simulink model "wrench_maats_simulator_v3"  (R2025b)
settings: Solver=ode15s  StartTime=0.0  StopTime=100  FixedStep=1e-4  RelTol=1e-3
values from neighbouring files (symbols this model uses):
  Kd1 = 2    [parametrosCarga4x.m]
  x1_0 = xL0+q1_rot*[0;0;L1]    [parametrosCarga4x.m]
  x2_0 = xL0+q2_rot*[0;0;L2]    [parametrosCarga4x.m]
  x3_0 = xL0+q3_rot*[0;0;L3]    [parametrosCarga4x.m]
  x4_0 = xL0+q4_rot*[0;0;L4]    [parametrosCarga4x.m]
settings Model: Creator=ateveraz  LastModifiedBy=ateveraz

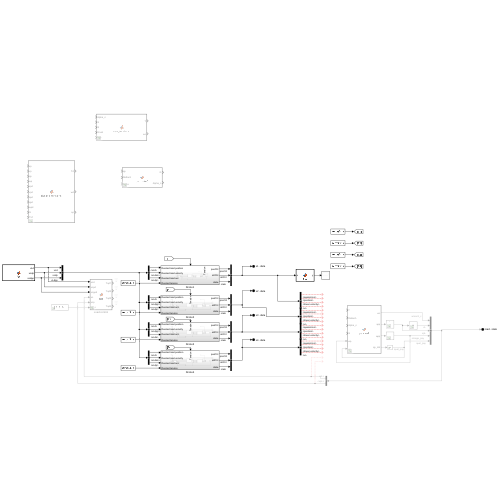
[thumbnail: Simulink's stored preview of the top-level diagram]
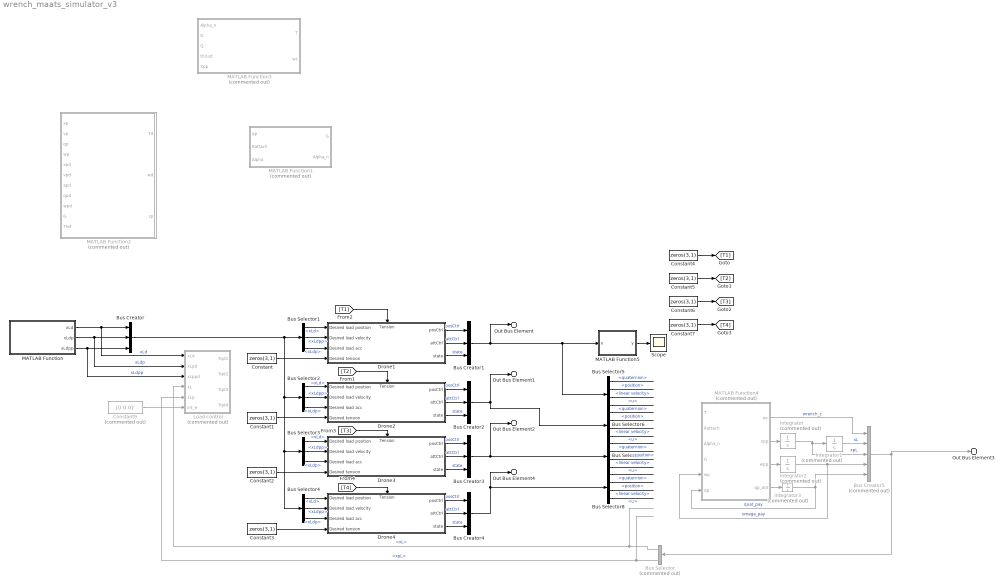
== system wrench_maats_simulator_v3 ==
  Bus Creator{,2..4} (4 alike) : BusCreator  Inputs=3
  Bus Creator1 : BusCreator  Inputs=3  OutDataTypeStr=Bus: busx1
  Bus Creator5 : BusCreator  Commented=on  Inputs=5
  Bus Selector : BusSelector  Commented=on  OutputSignals=xL,xpL
  Bus Selector{1..4} (4 alike) : BusSelector  OutputSignals=xLd,xLdpp,xLdp
  Bus Selector{5..8} (4 alike) : BusSelector  OutputSignals=state.quaternion,state.position,state.linear velocity,posCtrl.u
  Constant{,1..7} (8 alike) : Constant  Value=zeros(3,1)
  Constant9 : Constant  Commented=on  Value=[0 0 0]'
  Drone1 : Subsystem
      settings: PortSchema="{\"entries\":[{\"content\":{\"sides\":[{\"content\":{\"connectorIds\":[\"In1\",\"In2\",\"In3\",\"In4\"]},\"type\":\"ConnectorPlacement.EquallySpacedRectSide\",\"uuid\":\"21103dfc-7bbe-40e0-9fc6-037905f1ea97\"},{\"content\":{\"connectorIds\":[\"Out1\",\"Out2\",\"Out3\"],\"side\":\"RIGHT\"},\"type\":\"ConnectorPlacement.EquallySpacedRectSide\",\"uuid\":\"5db0cf3b-93f2-491f-9cf6-07daf4674486\"},{\"content\":{\"connectorIds\":[\"In5\"],\"side\":\"TOP\"},\"type\":\"ConnectorPlacement.EquallySpacedRectSide\",\"uuid\":\"a4b55797-f354-4dcd-9bd0-022aba8efa3f\"}]},\"type\":\"ConnectorPlacement.EquallySpacedConnector\",\"uuid\":\"4e7ed67a-de76-4120-bfce-551a78690751\"}],\"packageUris\":[\"http://schema.mathworks.com/mf0/Connector/R2020b\"],\"version\":\"1.0\"}"
  Drone2 : Subsystem
      settings: PortSchema="{\"entries\":[{\"content\":{\"sides\":[{\"content\":{\"connectorIds\":[\"In1\",\"In2\",\"In3\",\"In4\"]},\"type\":\"ConnectorPlacement.EquallySpacedRectSide\",\"uuid\":\"21103dfc-7bbe-40e0-9fc6-037905f1ea97\"},{\"content\":{\"connectorIds\":[\"Out1\",\"Out2\",\"Out3\"],\"side\":\"RIGHT\"},\"type\":\"ConnectorPlacement.EquallySpacedRectSide\",\"uuid\":\"5db0cf3b-93f2-491f-9cf6-07daf4674486\"},{\"content\":{\"connectorIds\":[\"In5\"],\"side\":\"TOP\"},\"type\":\"ConnectorPlacement.EquallySpacedRectSide\",\"uuid\":\"a4b55797-f354-4dcd-9bd0-022aba8efa3f\"}]},\"type\":\"ConnectorPlacement.EquallySpacedConnector\",\"uuid\":\"4e7ed67a-de76-4120-bfce-551a78690751\"}],\"packageUris\":[\"http://schema.mathworks.com/mf0/Connector/R2020b\"],\"version\":\"1.0\"}"
  Drone3 : Subsystem
      settings: PortSchema="{\"entries\":[{\"content\":{\"sides\":[{\"content\":{\"connectorIds\":[\"In1\",\"In2\",\"In3\",\"In4\"]},\"type\":\"ConnectorPlacement.EquallySpacedRectSide\",\"uuid\":\"21103dfc-7bbe-40e0-9fc6-037905f1ea97\"},{\"content\":{\"connectorIds\":[\"Out1\",\"Out2\",\"Out3\"],\"side\":\"RIGHT\"},\"type\":\"ConnectorPlacement.EquallySpacedRectSide\",\"uuid\":\"5db0cf3b-93f2-491f-9cf6-07daf4674486\"},{\"content\":{\"connectorIds\":[\"In5\"],\"side\":\"TOP\"},\"type\":\"ConnectorPlacement.EquallySpacedRectSide\",\"uuid\":\"a4b55797-f354-4dcd-9bd0-022aba8efa3f\"}]},\"type\":\"ConnectorPlacement.EquallySpacedConnector\",\"uuid\":\"4e7ed67a-de76-4120-bfce-551a78690751\"}],\"packageUris\":[\"http://schema.mathworks.com/mf0/Connector/R2020b\"],\"version\":\"1.0\"}"
  Drone4 : Subsystem
      settings: PortSchema="{\"entries\":[{\"content\":{\"sides\":[{\"content\":{\"connectorIds\":[\"In1\",\"In2\",\"In3\",\"In4\"]},\"type\":\"ConnectorPlacement.EquallySpacedRectSide\",\"uuid\":\"21103dfc-7bbe-40e0-9fc6-037905f1ea97\"},{\"content\":{\"connectorIds\":[\"Out1\",\"Out2\",\"Out3\"],\"side\":\"RIGHT\"},\"type\":\"ConnectorPlacement.EquallySpacedRectSide\",\"uuid\":\"5db0cf3b-93f2-491f-9cf6-07daf4674486\"},{\"content\":{\"connectorIds\":[\"In5\"],\"side\":\"TOP\"},\"type\":\"ConnectorPlacement.EquallySpacedRectSide\",\"uuid\":\"a4b55797-f354-4dcd-9bd0-022aba8efa3f\"}]},\"type\":\"ConnectorPlacement.EquallySpacedConnector\",\"uuid\":\"4e7ed67a-de76-4120-bfce-551a78690751\"}],\"packageUris\":[\"http://schema.mathworks.com/mf0/Connector/R2020b\"],\"version\":\"1.0\"}"
  Integrator{,1..3} (4 alike) : Integrator  Commented=on
  Load control : MATLAB Function  Commented=on  TreatAsAtomicUnit=on
  MATLAB Function : MATLAB Function  TreatAsAtomicUnit=on
  MATLAB Function1 : MATLAB Function  Commented=on  TreatAsAtomicUnit=on
  MATLAB Function2 : MATLAB Function  Commented=on  TreatAsAtomicUnit=on
  MATLAB Function3 : MATLAB Function  Commented=on  TreatAsAtomicUnit=on
  MATLAB Function4 : MATLAB Function  Commented=on  TreatAsAtomicUnit=on
  MATLAB Function5 : MATLAB Function  TreatAsAtomicUnit=on
  Scope : Scope
  Out Bus Element3 : Outport  PortName=load  Element=state
  Out Bus Element : Outport  Port=2  PortName=x1  Element=data
  Out Bus Element1 : Outport  Port=3  PortName=x2  Element=data
  Out Bus Element2 : Outport  Port=4  PortName=x3  Element=data
  Out Bus Element4 : Outport  Port=5  PortName=x4  Element=data
  wires:
  Drone1/1(posCtrl) -> Bus Creator1/1  "posCtrl"
  Drone1/2(attCtrl) -> Bus Creator1/2  "attCtrl"
  Drone1/3(state) -> Bus Creator1/3  "state"
  MATLAB Function/1(xLd) -> Load control/1(xLd), Bus Creator/1  "xLd"
  MATLAB Function/2(xLdp) -> Load control/2(xLpd), Bus Creator/2  "xLdp"
  MATLAB Function/3(xLdpp) -> Load control/3(xLppd), Bus Creator/3  "xLdpp"
  Constant9/1 -> Load control/6(int_e)
  Bus Creator5/1 -> Out Bus Element3/1, Bus Selector/1
  Bus Selector/2 -> Load control/5(xLp)  "<xpL>"
  Bus Selector/1 -> Load control/4(xL)  "<xL>"
  Bus Selector1/1 -> Drone1/1(Desired load position)  "<xLd>"
  Bus Selector1/2 -> Drone1/2(Desired load velocity)  "<xLdpp>"
  Bus Selector1/3 -> Drone1/3(Desired load acc)  "<xLdp>"
  Bus Selector2/3 -> Drone2/3(Desired load acc)  "<xLdp>"
  Bus Selector2/2 -> Drone2/2(Desired load velocity)  "<xLdpp>"
  Bus Selector2/1 -> Drone2/1(Desired load position)  "<xLd>"
  Bus Creator/1 -> Bus Selector4/1, Bus Selector3/1, Bus Selector2/1, Bus Selector1/1
  Bus Selector3/2 -> Drone3/2(Desired load velocity)  "<xLdpp>"
  Bus Selector3/3 -> Drone3/3(Desired load acc)  "<xLdp>"
  Bus Selector3/1 -> Drone3/1(Desired load position)  "<xLd>"
  Bus Selector4/1 -> Drone4/1(Desired load position)  "<xLd>"
  Bus Selector4/3 -> Drone4/3(Desired load acc)  "<xLdp>"
  Bus Selector4/2 -> Drone4/2(Desired load velocity)  "<xLdpp>"
  Bus Creator1/1 -> MATLAB Function5/1(u), Bus Selector5/1, Out Bus Element/1
  Bus Creator2/1 -> Out Bus Element1/1, Bus Selector6/1
  Drone2/3(state) -> Bus Creator2/3  "state"
  Drone2/2(attCtrl) -> Bus Creator2/2  "attCtrl"
  Drone2/1(posCtrl) -> Bus Creator2/1  "posCtrl"
  Drone3/1(posCtrl) -> Bus Creator3/1  "posCtrl"
  Drone3/2(attCtrl) -> Bus Creator3/2  "attCtrl"
  Drone3/3(state) -> Bus Creator3/3  "state"
  Bus Creator3/1 -> Out Bus Element2/1, Bus Selector7/1
  Bus Creator4/1 -> Bus Selector8/1, Out Bus Element4/1
  Drone4/3(state) -> Bus Creator4/3  "state"
  Drone4/2(attCtrl) -> Bus Creator4/2  "attCtrl"
  Drone4/1(posCtrl) -> Bus Creator4/1  "posCtrl"
  Bus Selector5/1 -> ?  "<quaternion>"
  Bus Selector5/2 -> ?  "<position>"
  Bus Selector5/3 -> ?  "<linear velocity>"
  Bus Selector5/4 -> ?  "<u>"
  Bus Selector6/1 -> ?  "<quaternion>"
  Bus Selector6/2 -> ?  "<position>"
  Bus Selector6/3 -> ?  "<linear velocity>"
  Bus Selector6/4 -> ?  "<u>"
  Bus Selector7/1 -> ?  "<quaternion>"
  Bus Selector7/2 -> ?  "<position>"
  Bus Selector7/3 -> ?  "<linear velocity>"
  Bus Selector7/4 -> ?  "<u>"
  Bus Selector8/1 -> ?  "<quaternion>"
  Bus Selector8/2 -> ?  "<position>"
  Bus Selector8/3 -> ?  "<linear velocity>"
  Bus Selector8/4 -> ?  "<u>"
  [T2] -> Drone2/5(Tension)
  [T3] -> Drone3/5(Tension)
  [T4] -> Drone4/5(Tension)
  [T1] -> Drone1/5(Tension)
  Integrator/1 -> Bus Creator5/3, Integrator1/1  "xpL"
  MATLAB Function4/3(wpp) -> Integrator2/1
  Integrator2/1 -> Bus Creator5/4, MATLAB Function4/5(wp)  "omega_pay"
  MATLAB Function4/4(qp_dot) -> Integrator3/1
  Integrator3/1 -> MATLAB Function4/6(qp), Bus Creator5/5  "quat_pay"
  MATLAB Function4/2(xpp) -> Integrator/1
  Integrator1/1 -> Bus Creator5/2  "xL"
  MATLAB Function4/1(wc) -> Bus Creator5/1  "wrench_c"
  Constant/1 -> Drone1/4(Desired tension)
  Constant1/1 -> Drone2/4(Desired tension)
  Constant2/1 -> Drone3/4(Desired tension)
  Constant3/1 -> Drone4/4(Desired tension)
  Constant4/1 -> [T1]
  Constant5/1 -> [T2]
  Constant6/1 -> [T3]
  Constant7/1 -> [T4]
  MATLAB Function5/1(y) -> Scope/1

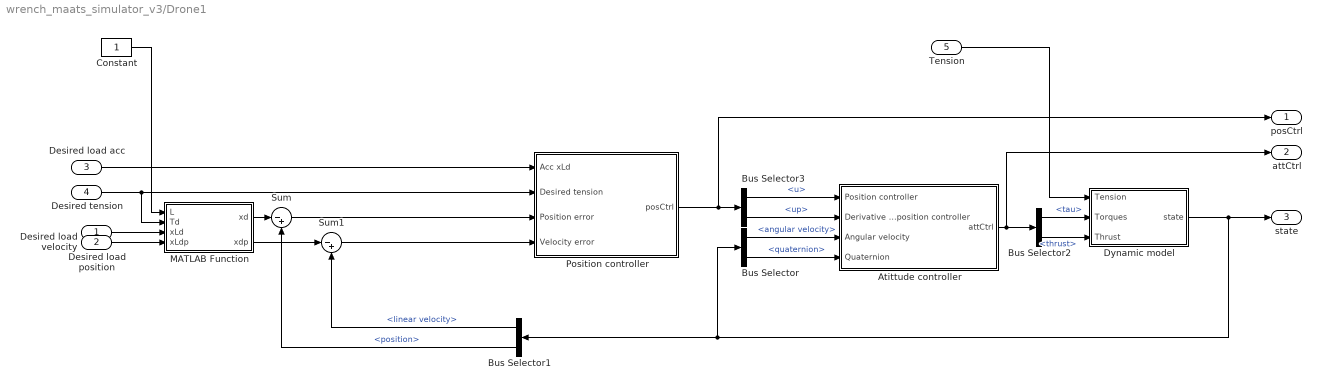
== system wrench_maats_simulator_v3/Drone1 ==
  Desired load position : Inport
  Desired load velocity : Inport  Port=2
  Desired load acc : Inport  Port=3
  Desired tension : Inport  Port=4
  Tension : Inport  Port=5
  Atittude controller : Subsystem
  Bus Selector : BusSelector  OutputSignals=angular velocity,quaternion
  Bus Selector1 : BusSelector  OutputSignals=linear velocity,position
  Bus Selector2 : BusSelector  OutputSignals=tau,thrust
  Bus Selector3 : BusSelector  OutputSignals=u,up
  Constant : Constant
  Dynamic model : Subsystem
  MATLAB Function : MATLAB Function  TreatAsAtomicUnit=on
  Position controller : Subsystem
  Sum : Sum  Inputs=|-+
  Sum1 : Sum  Inputs=|-+
  posCtrl : Outport
  attCtrl : Outport  Port=2
  state : Outport  Port=3
  wires:
  Sum1/1 -> Position controller/4(Velocity error)
  Desired load velocity/1 -> MATLAB Function/4(xLdp)
  Bus Selector3/1 -> Atittude controller/1(Position controller)  "<u>"
  Bus Selector2/1 -> Dynamic model/2(Torques)  "<tau>"
  Atittude controller/1(attCtrl) -> attCtrl/1, Bus Selector2/1
  Desired tension/1 -> MATLAB Function/2(Td), Position controller/2(Desired tension)
  Desired load acc/1 -> Position controller/1(Acc xLd)
  Sum/1 -> Position controller/3(Position error)
  Bus Selector1/2 -> Sum/2  "<position>"
  Position controller/1(posCtrl) -> posCtrl/1, Bus Selector3/1
  Bus Selector2/2 -> Dynamic model/3(Thrust)  "<thrust>"
  Desired load position/1 -> MATLAB Function/3(xLd)
  Bus Selector1/1 -> Sum1/2  "<linear velocity>"
  Dynamic model/1(state) -> Bus Selector/1, Bus Selector1/1, state/1
  Bus Selector3/2 -> Atittude controller/2(Derivative position controller)  "<up>"
  MATLAB Function/1(xd) -> Sum/1
  MATLAB Function/2(xdp) -> Sum1/1
  Constant/1 -> MATLAB Function/1(L)
  Tension/1 -> Dynamic model/1(Tension)
  Bus Selector/1 -> Atittude controller/3(Angular velocity)  "<angular velocity>"
  Bus Selector/2 -> Atittude controller/4(Quaternion)  "<quaternion>"

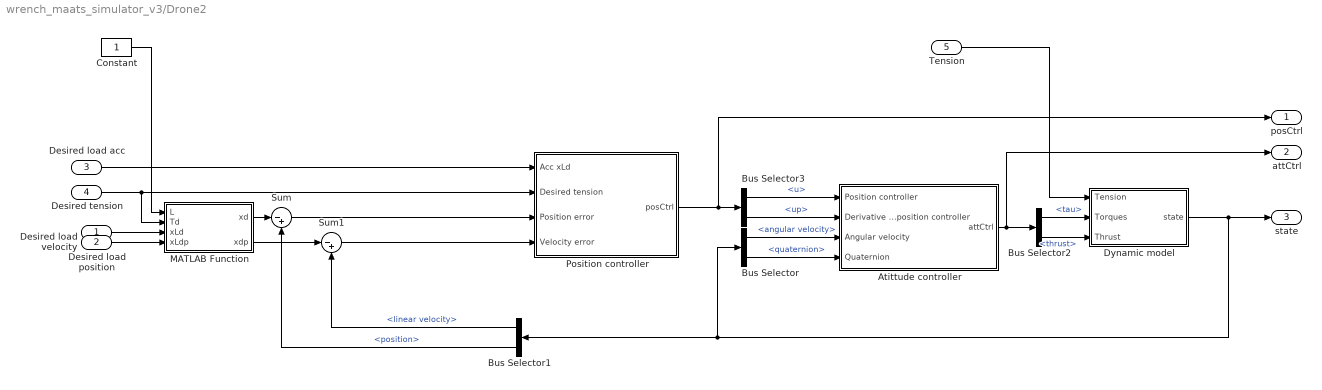
== system wrench_maats_simulator_v3/Drone2 ==
  Desired load position : Inport
  Desired load velocity : Inport  Port=2
  Desired load acc : Inport  Port=3
  Desired tension : Inport  Port=4
  Tension : Inport  Port=5
  Atittude controller : Subsystem
  Bus Selector : BusSelector  OutputSignals=angular velocity,quaternion
  Bus Selector1 : BusSelector  OutputSignals=linear velocity,position
  Bus Selector2 : BusSelector  OutputSignals=tau,thrust
  Bus Selector3 : BusSelector  OutputSignals=u,up
  Constant : Constant
  Dynamic model : Subsystem
  MATLAB Function : MATLAB Function  TreatAsAtomicUnit=on
  Position controller : Subsystem
  Sum : Sum  Inputs=|-+
  Sum1 : Sum  Inputs=|-+
  posCtrl : Outport
  attCtrl : Outport  Port=2
  state : Outport  Port=3
  wires:
  Bus Selector/2 -> Atittude controller/4(Quaternion)  "<quaternion>"
  Bus Selector/1 -> Atittude controller/3(Angular velocity)  "<angular velocity>"
  Tension/1 -> Dynamic model/1(Tension)
  Constant/1 -> MATLAB Function/1(L)
  MATLAB Function/2(xdp) -> Sum1/1
  MATLAB Function/1(xd) -> Sum/1
  Bus Selector3/2 -> Atittude controller/2(Derivative position controller)  "<up>"
  Dynamic model/1(state) -> state/1, Bus Selector1/1, Bus Selector/1
  Bus Selector1/1 -> Sum1/2  "<linear velocity>"
  Desired load position/1 -> MATLAB Function/3(xLd)
  Bus Selector2/2 -> Dynamic model/3(Thrust)  "<thrust>"
  Position controller/1(posCtrl) -> Bus Selector3/1, posCtrl/1
  Bus Selector1/2 -> Sum/2  "<position>"
  Sum/1 -> Position controller/3(Position error)
  Desired load acc/1 -> Position controller/1(Acc xLd)
  Desired tension/1 -> Position controller/2(Desired tension), MATLAB Function/2(Td)
  Atittude controller/1(attCtrl) -> Bus Selector2/1, attCtrl/1
  Bus Selector2/1 -> Dynamic model/2(Torques)  "<tau>"
  Bus Selector3/1 -> Atittude controller/1(Position controller)  "<u>"
  Desired load velocity/1 -> MATLAB Function/4(xLdp)
  Sum1/1 -> Position controller/4(Velocity error)

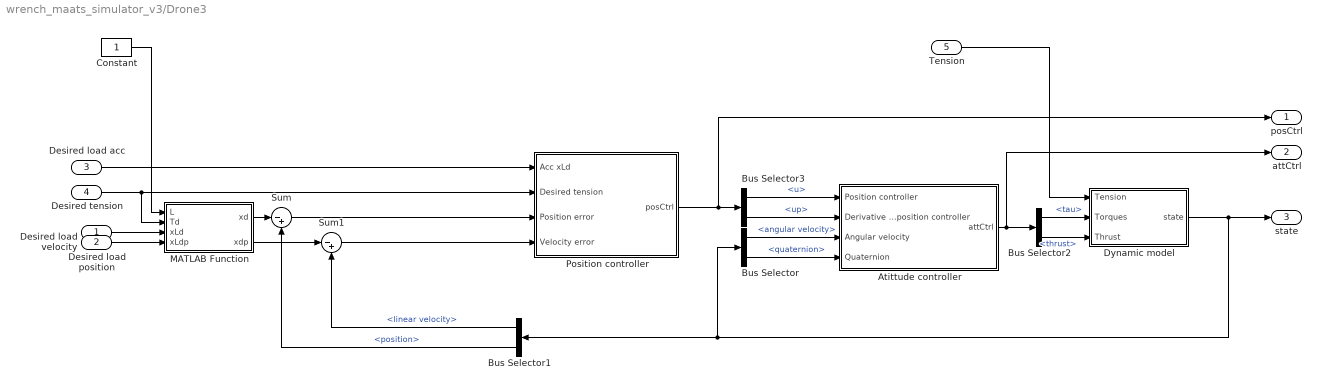
== system wrench_maats_simulator_v3/Drone3 ==
  Desired load position : Inport
  Desired load velocity : Inport  Port=2
  Desired load acc : Inport  Port=3
  Desired tension : Inport  Port=4
  Tension : Inport  Port=5
  Atittude controller : Subsystem
  Bus Selector : BusSelector  OutputSignals=angular velocity,quaternion
  Bus Selector1 : BusSelector  OutputSignals=linear velocity,position
  Bus Selector2 : BusSelector  OutputSignals=tau,thrust
  Bus Selector3 : BusSelector  OutputSignals=u,up
  Constant : Constant
  Dynamic model : Subsystem
  MATLAB Function : MATLAB Function  TreatAsAtomicUnit=on
  Position controller : Subsystem
  Sum : Sum  Inputs=|-+
  Sum1 : Sum  Inputs=|-+
  posCtrl : Outport
  attCtrl : Outport  Port=2
  state : Outport  Port=3
  wires:
  Sum1/1 -> Position controller/4(Velocity error)
  Desired load velocity/1 -> MATLAB Function/4(xLdp)
  Bus Selector3/1 -> Atittude controller/1(Position controller)  "<u>"
  Bus Selector2/1 -> Dynamic model/2(Torques)  "<tau>"
  Atittude controller/1(attCtrl) -> attCtrl/1, Bus Selector2/1
  Desired tension/1 -> MATLAB Function/2(Td), Position controller/2(Desired tension)
  Desired load acc/1 -> Position controller/1(Acc xLd)
  Sum/1 -> Position controller/3(Position error)
  Bus Selector1/2 -> Sum/2  "<position>"
  Position controller/1(posCtrl) -> posCtrl/1, Bus Selector3/1
  Bus Selector2/2 -> Dynamic model/3(Thrust)  "<thrust>"
  Desired load position/1 -> MATLAB Function/3(xLd)
  Bus Selector1/1 -> Sum1/2  "<linear velocity>"
  Dynamic model/1(state) -> Bus Selector/1, Bus Selector1/1, state/1
  Bus Selector3/2 -> Atittude controller/2(Derivative position controller)  "<up>"
  MATLAB Function/1(xd) -> Sum/1
  MATLAB Function/2(xdp) -> Sum1/1
  Constant/1 -> MATLAB Function/1(L)
  Tension/1 -> Dynamic model/1(Tension)
  Bus Selector/1 -> Atittude controller/3(Angular velocity)  "<angular velocity>"
  Bus Selector/2 -> Atittude controller/4(Quaternion)  "<quaternion>"

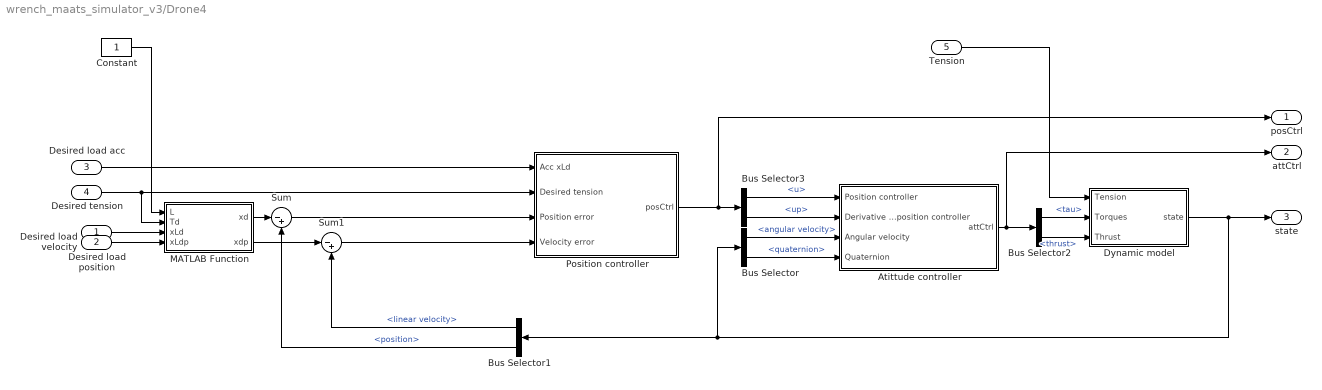
== system wrench_maats_simulator_v3/Drone4 ==
  Desired load position : Inport
  Desired load velocity : Inport  Port=2
  Desired load acc : Inport  Port=3
  Desired tension : Inport  Port=4
  Tension : Inport  Port=5
  Atittude controller : Subsystem
  Bus Selector : BusSelector  OutputSignals=angular velocity,quaternion
  Bus Selector1 : BusSelector  OutputSignals=linear velocity,position
  Bus Selector2 : BusSelector  OutputSignals=tau,thrust
  Bus Selector3 : BusSelector  OutputSignals=u,up
  Constant : Constant
  Dynamic model : Subsystem
  MATLAB Function : MATLAB Function  TreatAsAtomicUnit=on
  Position controller : Subsystem
  Sum : Sum  Inputs=|-+
  Sum1 : Sum  Inputs=|-+
  posCtrl : Outport
  attCtrl : Outport  Port=2
  state : Outport  Port=3
  wires:
  Bus Selector/2 -> Atittude controller/4(Quaternion)  "<quaternion>"
  Bus Selector/1 -> Atittude controller/3(Angular velocity)  "<angular velocity>"
  Tension/1 -> Dynamic model/1(Tension)
  Constant/1 -> MATLAB Function/1(L)
  MATLAB Function/2(xdp) -> Sum1/1
  MATLAB Function/1(xd) -> Sum/1
  Bus Selector3/2 -> Atittude controller/2(Derivative position controller)  "<up>"
  Dynamic model/1(state) -> state/1, Bus Selector1/1, Bus Selector/1
  Bus Selector1/1 -> Sum1/2  "<linear velocity>"
  Desired load position/1 -> MATLAB Function/3(xLd)
  Bus Selector2/2 -> Dynamic model/3(Thrust)  "<thrust>"
  Position controller/1(posCtrl) -> Bus Selector3/1, posCtrl/1
  Bus Selector1/2 -> Sum/2  "<position>"
  Sum/1 -> Position controller/3(Position error)
  Desired load acc/1 -> Position controller/1(Acc xLd)
  Desired tension/1 -> Position controller/2(Desired tension), MATLAB Function/2(Td)
  Atittude controller/1(attCtrl) -> Bus Selector2/1, attCtrl/1
  Bus Selector2/1 -> Dynamic model/2(Torques)  "<tau>"
  Bus Selector3/1 -> Atittude controller/1(Position controller)  "<u>"
  Desired load velocity/1 -> MATLAB Function/4(xLdp)
  Sum1/1 -> Position controller/4(Velocity error)

== system wrench_maats_simulator_v3/Drone1/Atittude controller ==
  Position controller : Inport
  Derivative position controller : Inport  Port=2
  Angular velocity : Inport  Port=3
  Quaternion : Inport  Port=4
  Bus Creator : BusCreator  Inputs=3
  MATLAB System1 : MATLABSystem  System=AttitudeController  Kd=1  beta=0.3  gamma=10  rho=18  SimulateUsing=Code generation
      mask Type: AttitudeController
  MATLAB System2 : MATLABSystem  System=DesiredAttitude  SimulateUsing=Code generation
      mask Type: DesiredAttitude
  attCtrl : Outport
  wires:
  Angular velocity/1 -> MATLAB System2/3
  MATLAB System2/2 -> MATLAB System1/3
  Position controller/1 -> MATLAB System1/1, MATLAB System2/1
  Quaternion/1 -> MATLAB System2/4
  MATLAB System2/1 -> Bus Creator/3, MATLAB System1/2  "error quaternion"
  Derivative position controller/1 -> MATLAB System2/2
  MATLAB System1/2 -> Bus Creator/2  "thrust"
  Bus Creator/1 -> attCtrl/1
  MATLAB System1/1 -> Bus Creator/1  "tau"

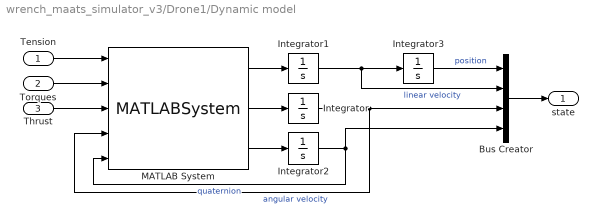
== system wrench_maats_simulator_v3/Drone1/Dynamic model ==
  Tension : Inport
  Torques : Inport  Port=2
  Thrust : Inport  Port=3
  Bus Creator : BusCreator  Inputs=4
  Integrator : Integrator  InitialCondition=[0 0 0]'
  Integrator1 : Integrator  InitialCondition=[0 0 0]'
  Integrator2 : Integrator  InitialCondition=[1 0 0 0]'
  Integrator3 : Integrator  InitialCondition=x1_0
  MATLAB System : MATLABSystem  System=Modelx4  mass=mi  inertia_matrix=J  SimulateUsing=Code generation
      mask Type: Modelx4
  state : Outport
  wires:
  MATLAB System/1 -> Integrator1/1
  Integrator3/1 -> Bus Creator/1  "position"
  MATLAB System/3 -> Integrator2/1
  MATLAB System/2 -> Integrator/1
  Integrator2/1 -> MATLAB System/5, Bus Creator/4  "quaternion"
  Torques/1 -> MATLAB System/2
  Integrator1/1 -> Bus Creator/2, Integrator3/1  "linear velocity"
  Thrust/1 -> MATLAB System/3
  Integrator/1 -> MATLAB System/4, Bus Creator/3  "angular velocity"
  Bus Creator/1 -> state/1
  Tension/1 -> MATLAB System/1

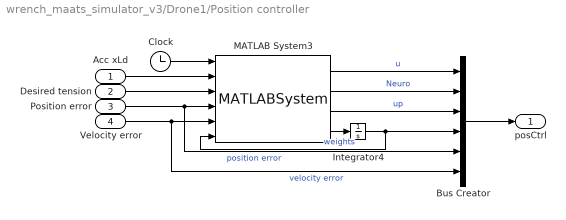
== system wrench_maats_simulator_v3/Drone1/Position controller ==
  Acc xLd : Inport
  Desired tension : Inport  Port=2
  Position error : Inport  Port=3
  Velocity error : Inport  Port=4
  Bus Creator : BusCreator  Inputs=6
  Clock : Clock
  Integrator4 : Integrator  InitialCondition=zeros(3,15)
  MATLAB System3 : MATLABSystem  System=PositionController  Kd=Kd1  alpha=Alpha1  mass=mi  Gamma=Gamma1  kappa=2  k=10  N_neurons=15  center_range=1  eta_width=linspace(1,10,15)  SimulateUsing=Interpreted execution
      mask Type: PositionController
  posCtrl : Outport
  wires:
  Position error/1 -> MATLAB System3/4, Bus Creator/5  "position error"
  Integrator4/1 -> MATLAB System3/6, Bus Creator/4  "weights"
  Bus Creator/1 -> posCtrl/1
  Velocity error/1 -> MATLAB System3/5, Bus Creator/6  "velocity error"
  MATLAB System3/4 -> Integrator4/1
  MATLAB System3/1 -> Bus Creator/1  "u"
  MATLAB System3/2 -> Bus Creator/2  "Neuro"
  MATLAB System3/3 -> Bus Creator/3  "up"
  Clock/1 -> MATLAB System3/1
  Acc xLd/1 -> MATLAB System3/2
  Desired tension/1 -> MATLAB System3/3

== system wrench_maats_simulator_v3/Drone2/Atittude controller ==
  Position controller : Inport
  Derivative position controller : Inport  Port=2
  Angular velocity : Inport  Port=3
  Quaternion : Inport  Port=4
  Bus Creator : BusCreator  Inputs=3
  MATLAB System1 : MATLABSystem  System=AttitudeController  Kd=1  beta=0.3  gamma=10  rho=18  SimulateUsing=Code generation
      mask Type: AttitudeController
  MATLAB System2 : MATLABSystem  System=DesiredAttitude  SimulateUsing=Code generation
      mask Type: DesiredAttitude
  attCtrl : Outport
  wires:
  MATLAB System1/1 -> Bus Creator/1  "tau"
  Bus Creator/1 -> attCtrl/1
  MATLAB System1/2 -> Bus Creator/2  "thrust"
  Derivative position controller/1 -> MATLAB System2/2
  MATLAB System2/1 -> MATLAB System1/2, Bus Creator/3  "error quaternion"
  Quaternion/1 -> MATLAB System2/4
  Position controller/1 -> MATLAB System2/1, MATLAB System1/1
  MATLAB System2/2 -> MATLAB System1/3
  Angular velocity/1 -> MATLAB System2/3

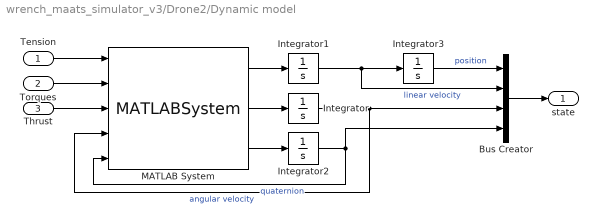
== system wrench_maats_simulator_v3/Drone2/Dynamic model ==
  Tension : Inport
  Torques : Inport  Port=2
  Thrust : Inport  Port=3
  Bus Creator : BusCreator  Inputs=4
  Integrator : Integrator  InitialCondition=[0 0 0]'
  Integrator1 : Integrator  InitialCondition=[0 0 0]'
  Integrator2 : Integrator  InitialCondition=[1 0 0 0]'
  Integrator3 : Integrator  InitialCondition=x2_0
  MATLAB System : MATLABSystem  System=Modelx4  mass=mi  inertia_matrix=J  SimulateUsing=Code generation
      mask Type: Modelx4
  state : Outport
  wires:
  Tension/1 -> MATLAB System/1
  Bus Creator/1 -> state/1
  Integrator/1 -> Bus Creator/3, MATLAB System/4  "angular velocity"
  Thrust/1 -> MATLAB System/3
  Integrator1/1 -> Integrator3/1, Bus Creator/2  "linear velocity"
  Torques/1 -> MATLAB System/2
  Integrator2/1 -> Bus Creator/4, MATLAB System/5  "quaternion"
  MATLAB System/2 -> Integrator/1
  MATLAB System/3 -> Integrator2/1
  Integrator3/1 -> Bus Creator/1  "position"
  MATLAB System/1 -> Integrator1/1

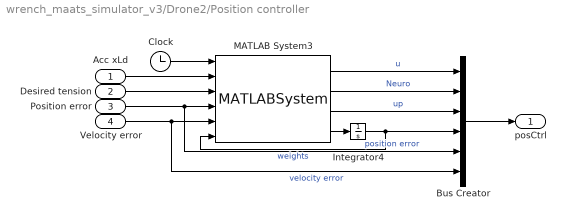
== system wrench_maats_simulator_v3/Drone2/Position controller ==
  Acc xLd : Inport
  Desired tension : Inport  Port=2
  Position error : Inport  Port=3
  Velocity error : Inport  Port=4
  Bus Creator : BusCreator  Inputs=6
  Clock : Clock
  Integrator4 : Integrator  InitialCondition=zeros(3,15)
  MATLAB System3 : MATLABSystem  System=PositionController  Kd=Kd1  alpha=Alpha1  mass=mi  Gamma=Gamma1  kappa=2  k=10  N_neurons=15  center_range=1  eta_width=linspace(1,10,15)  SimulateUsing=Interpreted execution
      mask Type: PositionController
  posCtrl : Outport
  wires:
  Desired tension/1 -> MATLAB System3/3
  Acc xLd/1 -> MATLAB System3/2
  Clock/1 -> MATLAB System3/1
  MATLAB System3/3 -> Bus Creator/3  "up"
  MATLAB System3/2 -> Bus Creator/2  "Neuro"
  MATLAB System3/1 -> Bus Creator/1  "u"
  MATLAB System3/4 -> Integrator4/1
  Velocity error/1 -> Bus Creator/6, MATLAB System3/5  "velocity error"
  Bus Creator/1 -> posCtrl/1
  Integrator4/1 -> Bus Creator/4, MATLAB System3/6  "weights"
  Position error/1 -> Bus Creator/5, MATLAB System3/4  "position error"

== system wrench_maats_simulator_v3/Drone3/Atittude controller ==
  Position controller : Inport
  Derivative position controller : Inport  Port=2
  Angular velocity : Inport  Port=3
  Quaternion : Inport  Port=4
  Bus Creator : BusCreator  Inputs=3
  MATLAB System1 : MATLABSystem  System=AttitudeController  Kd=1  beta=0.3  gamma=10  rho=18  SimulateUsing=Code generation
      mask Type: AttitudeController
  MATLAB System2 : MATLABSystem  System=DesiredAttitude  SimulateUsing=Code generation
      mask Type: DesiredAttitude
  attCtrl : Outport
  wires:
  Angular velocity/1 -> MATLAB System2/3
  MATLAB System2/2 -> MATLAB System1/3
  Position controller/1 -> MATLAB System1/1, MATLAB System2/1
  Quaternion/1 -> MATLAB System2/4
  MATLAB System2/1 -> Bus Creator/3, MATLAB System1/2  "error quaternion"
  Derivative position controller/1 -> MATLAB System2/2
  MATLAB System1/2 -> Bus Creator/2  "thrust"
  Bus Creator/1 -> attCtrl/1
  MATLAB System1/1 -> Bus Creator/1  "tau"

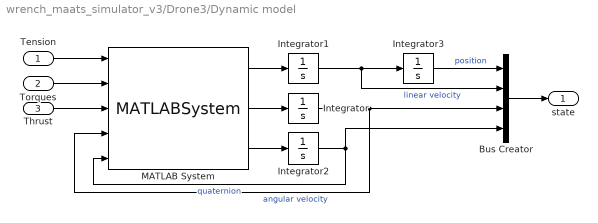
== system wrench_maats_simulator_v3/Drone3/Dynamic model ==
  Tension : Inport
  Torques : Inport  Port=2
  Thrust : Inport  Port=3
  Bus Creator : BusCreator  Inputs=4
  Integrator : Integrator  InitialCondition=[0 0 0]'
  Integrator1 : Integrator  InitialCondition=[0 0 0]'
  Integrator2 : Integrator  InitialCondition=[1 0 0 0]'
  Integrator3 : Integrator  InitialCondition=x3_0
  MATLAB System : MATLABSystem  System=Modelx4  mass=mi  inertia_matrix=J  SimulateUsing=Code generation
      mask Type: Modelx4
  state : Outport
  wires:
  MATLAB System/1 -> Integrator1/1
  Integrator3/1 -> Bus Creator/1  "position"
  MATLAB System/3 -> Integrator2/1
  MATLAB System/2 -> Integrator/1
  Integrator2/1 -> MATLAB System/5, Bus Creator/4  "quaternion"
  Torques/1 -> MATLAB System/2
  Integrator1/1 -> Bus Creator/2, Integrator3/1  "linear velocity"
  Thrust/1 -> MATLAB System/3
  Integrator/1 -> MATLAB System/4, Bus Creator/3  "angular velocity"
  Bus Creator/1 -> state/1
  Tension/1 -> MATLAB System/1

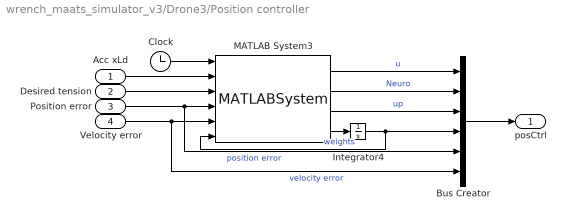
== system wrench_maats_simulator_v3/Drone3/Position controller ==
  Acc xLd : Inport
  Desired tension : Inport  Port=2
  Position error : Inport  Port=3
  Velocity error : Inport  Port=4
  Bus Creator : BusCreator  Inputs=6
  Clock : Clock
  Integrator4 : Integrator  InitialCondition=zeros(3,15)
  MATLAB System3 : MATLABSystem  System=PositionController  Kd=Kd1  alpha=Alpha1  mass=mi  Gamma=Gamma1  kappa=2  k=10  N_neurons=15  center_range=1  eta_width=linspace(1,10,15)  SimulateUsing=Interpreted execution
      mask Type: PositionController
  posCtrl : Outport
  wires:
  Position error/1 -> MATLAB System3/4, Bus Creator/5  "position error"
  Integrator4/1 -> MATLAB System3/6, Bus Creator/4  "weights"
  Bus Creator/1 -> posCtrl/1
  Velocity error/1 -> MATLAB System3/5, Bus Creator/6  "velocity error"
  MATLAB System3/4 -> Integrator4/1
  MATLAB System3/1 -> Bus Creator/1  "u"
  MATLAB System3/2 -> Bus Creator/2  "Neuro"
  MATLAB System3/3 -> Bus Creator/3  "up"
  Clock/1 -> MATLAB System3/1
  Acc xLd/1 -> MATLAB System3/2
  Desired tension/1 -> MATLAB System3/3

== system wrench_maats_simulator_v3/Drone4/Atittude controller ==
  Position controller : Inport
  Derivative position controller : Inport  Port=2
  Angular velocity : Inport  Port=3
  Quaternion : Inport  Port=4
  Bus Creator : BusCreator  Inputs=3
  MATLAB System1 : MATLABSystem  System=AttitudeController  Kd=1  beta=0.3  gamma=10  rho=18  SimulateUsing=Code generation
      mask Type: AttitudeController
  MATLAB System2 : MATLABSystem  System=DesiredAttitude  SimulateUsing=Code generation
      mask Type: DesiredAttitude
  attCtrl : Outport
  wires:
  MATLAB System1/1 -> Bus Creator/1  "tau"
  Bus Creator/1 -> attCtrl/1
  MATLAB System1/2 -> Bus Creator/2  "thrust"
  Derivative position controller/1 -> MATLAB System2/2
  MATLAB System2/1 -> MATLAB System1/2, Bus Creator/3  "error quaternion"
  Quaternion/1 -> MATLAB System2/4
  Position controller/1 -> MATLAB System2/1, MATLAB System1/1
  MATLAB System2/2 -> MATLAB System1/3
  Angular velocity/1 -> MATLAB System2/3

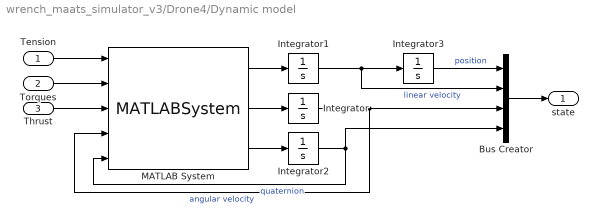
== system wrench_maats_simulator_v3/Drone4/Dynamic model ==
  Tension : Inport
  Torques : Inport  Port=2
  Thrust : Inport  Port=3
  Bus Creator : BusCreator  Inputs=4
  Integrator : Integrator  InitialCondition=[0 0 0]'
  Integrator1 : Integrator  InitialCondition=[0 0 0]'
  Integrator2 : Integrator  InitialCondition=[1 0 0 0]'
  Integrator3 : Integrator  InitialCondition=x4_0
  MATLAB System : MATLABSystem  System=Modelx4  mass=mi  inertia_matrix=J  SimulateUsing=Code generation
      mask Type: Modelx4
  state : Outport
  wires:
  Tension/1 -> MATLAB System/1
  Bus Creator/1 -> state/1
  Integrator/1 -> Bus Creator/3, MATLAB System/4  "angular velocity"
  Thrust/1 -> MATLAB System/3
  Integrator1/1 -> Integrator3/1, Bus Creator/2  "linear velocity"
  Torques/1 -> MATLAB System/2
  Integrator2/1 -> Bus Creator/4, MATLAB System/5  "quaternion"
  MATLAB System/2 -> Integrator/1
  MATLAB System/3 -> Integrator2/1
  Integrator3/1 -> Bus Creator/1  "position"
  MATLAB System/1 -> Integrator1/1

== system wrench_maats_simulator_v3/Drone4/Position controller ==
  Acc xLd : Inport
  Desired tension : Inport  Port=2
  Position error : Inport  Port=3
  Velocity error : Inport  Port=4
  Bus Creator : BusCreator  Inputs=6
  Clock : Clock
  Integrator4 : Integrator  InitialCondition=zeros(3,15)
  MATLAB System3 : MATLABSystem  System=PositionController  Kd=Kd1  alpha=Alpha1  mass=mi  Gamma=Gamma1  kappa=2  k=10  N_neurons=15  center_range=1  eta_width=linspace(1,10,15)  SimulateUsing=Interpreted execution
      mask Type: PositionController
  posCtrl : Outport
  wires:
  Desired tension/1 -> MATLAB System3/3
  Acc xLd/1 -> MATLAB System3/2
  Clock/1 -> MATLAB System3/1
  MATLAB System3/3 -> Bus Creator/3  "up"
  MATLAB System3/2 -> Bus Creator/2  "Neuro"
  MATLAB System3/1 -> Bus Creator/1  "u"
  MATLAB System3/4 -> Integrator4/1
  Velocity error/1 -> Bus Creator/6, MATLAB System3/5  "velocity error"
  Bus Creator/1 -> posCtrl/1
  Integrator4/1 -> Bus Creator/4, MATLAB System3/6  "weights"
  Position error/1 -> Bus Creator/5, MATLAB System3/4  "position error"

== matlab function wrench_maats_simulator_v3/MATLAB Function3 ==
  data: Alpha_n input; T output; G input; Q input; thrust input; Xpp input; wc output
function [T, wc] = real_tensions(Alpha_n, G, Q, thrust, Xpp)
%#codegen
% Alpha_n : 3xn
% G       : 6xn
% Q       : 4xn
% thrust  : nx1
% Xpp     : 3xn

mi = 0.4;   % si todos los UAVs tienen la misma masa
g  = 9.81;
ez = [0;0;1];

n = size(Alpha_n,2);
T = zeros(n,1);

for i = 1:n
    ui = thrust(i) * rotate_by_quat(Q(:,i), ez);
    Ti = Alpha_n(:,i).' * (mi * Xpp(:,i) + ui - mi * g * ez);

    if Ti < 0
        Ti = 0;
    end
    T(i) = Ti;
end

wc = G * T;

end

%% ===== Helpers =====
function vI = rotate_by_quat(q, v)
vq = [0; v];
tmp = quat_mult(q, vq);
tmp = quat_mult(tmp, quat_conj(q));
vI = tmp(2:4);
end

function q = quat_conj(qin)
q = [qin(1); -qin(2:4)];
end

function q = quat_mult(p,r)
q = [ p(1)*r(1) - p(2:4).'*r(2:4);
      p(1)*r(2:4) + r(1)*p(2:4) + cross(p(2:4),r(2:4)) ];
end

== matlab function wrench_maats_simulator_v3/MATLAB Function4 ==
  data: wc output; T input; Rattach input; Alpha_n input; G input; wp input; qp input; xpp output; wpp output; qp_dot output
function [wc, xpp, wpp, qp_dot] = payload(T, Rattach, Alpha_n, G, wp, qp)
%#codegen
% qp      : 4x1  (quaternion del payload)
% wp      : 3x1  (velocidad angular en P)
% T       : nx1  (tensiones reales)
% Rattach : 3xn  (puntos de anclaje en P)
% Alpha_n : 3xn  (direcciones de cable en I, normalizadas)
% G       : 6xn  (matriz geométrica de cables)

mp = 0.225;
Jp = diag([0.01 0.01 0.02]);   % ajusta con tu carga real
g  = 9.81;
ez = [0;0;1];

hp = zeros(3,1);   % disturbios translacionales (por ahora 0)
gp = zeros(3,1);   % disturbios rotacionales (por ahora 0)

n = size(Alpha_n,2);

%% Translational dynamics: mp ẍp = mp g ez - sum Ti alpha_i + hp
sumTa = zeros(3,1);
for i = 1:n
    sumTa = sumTa + T(i) * Alpha_n(:,i);
end

xpp = g * ez - (1/mp) * sumTa + hp/mp;

%% Rotational dynamics: Jp ω̇p = Σ r_i × f_i - ωp×Jp ωp + gp
Mp_cables = zeros(3,1);
for i = 1:n
    fiP = rotate_by_quat_conj(qp, T(i) * Alpha_n(:,i)); % fuerza en P
    Mp_cables = Mp_cables + cross(Rattach(:,i), fiP);
end

wpp = Jp \ (Mp_cables - cross(wp, Jp*wp) + gp);

%% Quaternion kinematics: q̇p = 0.5 * qp ⊗ <ωp>_Q
omega_q = [0; wp];            % pure quaternion de ωp
qp_dot  = 0.5 * quat_mult(qp, omega_q);

%% Wrench from cable geometry
wc = G * T;

end

%% ===== Helpers =====
function vR = rotate_by_quat_conj(q, v)
qc = quat_conj(q);
vq = [0; v];
tmp = quat_mult(qc, vq);
tmp = quat_mult(tmp, q);
vR = tmp(2:4);
end

function q = quat_conj(qin)
q = [qin(1); -qin(2:4)];
end

function q = quat_mult(p,r)
q = [ p(1)*r(1) - p(2:4).'*r(2:4);
      p(1)*r(2:4) + r(1)*p(2:4) + cross(p(2:4),r(2:4)) ];
end

== matlab function wrench_maats_simulator_v3/MATLAB Function5 ==
  data: u input Bus: busx1; y output
function y = fcn(u)
    y = u.state.quaternion;
end

== matlab function wrench_maats_simulator_v3/Load control ==
  data: xLd input; xLpd input; xLppd input; xL input; xLp input; Tqd1 output; Tqd2 output; Tqd3 output; int_e input; Tqd4 output
function [Tqd1,Tqd2,Tqd3,Tqd4] = fcn(xLd,xLpd,xLppd,xL,xLp,int_e)
    mL = 0.225;
    g  = [0;0;9.81];

    kpl = 1*diag([1,1,1]);
    kdl = 0.5*diag([1,1,1]);
    kil = 0*diag([1,1,1]);

    % Control de carga: fuerza deseada uL (como en el paper)
    uL = - mL * (g + xLppd) ...
         - kpl * (xL - xLd) ...
         - kdl * (xLp - xLpd) ...
         - kil * int_e;

    % Tensiones base en geometría de 4 drones
    Tqd2 = -(mL/4) * rotz(65)  * roty(-35) * g;
    Tqd3 = -(mL/4) * rotz(155) * roty(-35) * g;
    Tqd4 = -(mL/4) * rotz(245) * roty(-35) * g;

    % Agente residual: suma de tensiones = -uL
    Tqd1 = uL - (Tqd2 + Tqd3 + Tqd4);
end

== matlab function wrench_maats_simulator_v3/MATLAB Function ==
  data: xLd output; xLdp output; xLdpp output
function [xLd, xLdp, xLdpp] = fcn()
    xLd = [1 1 0]';
    xLdp = zeros(3,1);
    xLdpp = zeros(3,1);
end

== matlab function wrench_maats_simulator_v3/Drone1/MATLAB Function ==
  data: L input; xd output; Td input; xLd input; xLdp input; xdp output
function [xd, xdp] = fcn(L,  Td, xLd, xLdp)
    alpha = zeros(3,1);
    if (norm(Td)~=0)
        alpha = Td/norm(Td);
    end
    xd = xLd - L*alpha;
    xdp = xLdp;
end

== matlab function wrench_maats_simulator_v3/Drone2/MATLAB Function ==
  data: L input; xd output; Td input; xLd input; xLdp input; xdp output
function [xd, xdp] = fcn(L,  Td, xLd, xLdp)
    alpha = zeros(3,1);
    if (norm(Td)~=0)
        alpha = Td/norm(Td);
    end
    xd = xLd - L*alpha;
    xdp = xLdp;
end

== matlab function wrench_maats_simulator_v3/Drone3/MATLAB Function ==
  data: L input; xd output; Td input; xLd input; xLdp input; xdp output
function [xd, xdp] = fcn(L,  Td, xLd, xLdp)
    alpha = zeros(3,1);
    if (norm(Td)~=0)
        alpha = Td/norm(Td);
    end
    xd = xLd - L*alpha;
    xdp = xLdp;
end

== matlab function wrench_maats_simulator_v3/Drone4/MATLAB Function ==
  data: L input; xd output; Td input; xLd input; xLdp input; xdp output
function [xd, xdp] = fcn(L,  Td, xLd, xLdp)
    alpha = zeros(3,1);
    if (norm(Td)~=0)
        alpha = Td/norm(Td);
    end
    xd = xLd - L*alpha;
    xdp = xLdp;
end

== matlab function wrench_maats_simulator_v3/MATLAB Function1 ==
  data: qp input; G output; Rattach input; Alpha input; Alpha_n output
function [G, Alpha_n] = computeG(qp, Rattach, Alpha)
%#codegen
% qp      : 4x1
% Rattach : 3xn
% Alpha   : 3xn

n = size(Alpha,2);
Alpha_n = zeros(3,n);
G = zeros(6,n);

for i = 1:n
    Alpha_n(:,i) = safe_unit(Alpha(:,i));
    aiP = rotate_by_quat_conj(qp, Alpha_n(:,i));

    G(:,i) = [ -Alpha_n(:,i);
                cross(Rattach(:,i), aiP) ];
end

end

%% ===== Helpers =====
function vR = rotate_by_quat_conj(q, v)
qc = quat_conj(q);
vq = [0; v];
tmp = quat_mult(qc, vq);
tmp = quat_mult(tmp, q);
vR = tmp(2:4);
end

function q = quat_conj(qin)
q = [qin(1); -qin(2:4)];
end

function q = quat_mult(p,r)
q = [ p(1)*r(1) - p(2:4).'*r(2:4);
      p(1)*r(2:4) + r(1)*p(2:4) + cross(p(2:4),r(2:4)) ];
end

function u = safe_unit(v)
n = norm(v);
if n < 1e-8
    u = [0;0;1];
else
    u = v/n;
end
end

== matlab function wrench_maats_simulator_v3/MATLAB Function2 ==
  data: xp input; Td output; vp input; qp input; wp input; xpd input; vpd input; apd input; qpd input; wpd input; G input; Tref input; wd output; sp output
function [Td, wd, sp] = desired_tensions( ...
    xp, vp, qp, wp, ...
    xpd, vpd, apd, qpd, wpd, ...
    G, Tref)
%#codegen
% xp,vp,xpd,vpd,apd,wp,wpd : 3x1
% qp,qpd : 4x1
% G      : 6xn
% Tref   : nx1

%% Parameters
mp = 0.225;
g  = 9.81;
ez = [0;0;1];

Lambda_x = diag([1.5 1.5 1.5]);
Lambda_R = diag([2.0 2.0 2.0]);
Ks       = diag([8 8 8 4 4 4]);

rhoT     = 1e-3;
rhoDelta = 1e-2;
Tmin     = 0.01;

n = size(G,2);

%% Quaternion error q_tilde = qd* \otimes q
qpd_conj = quat_conj(qpd);
qtilde   = quat_mult(qpd_conj, qp);
if qtilde(1) < 0
    qtilde = -qtilde;
end

%% Payload manifold
xtilde = xp - xpd;
vtilde = vp - vpd;
wtilde = wp - wpd;

sx = vtilde + Lambda_x * xtilde;
sR = wtilde + Lambda_R * qtilde(2:4);
sp = [sx; sR];

%% Wrench-feasible projection
PG = G * pinv(G);

%% Feedforward wrench
wff = [mp*apd + mp*g*ez;
       zeros(3,1)];

%% Desired wrench without NN
wd = -Ks * (PG * sp) + wff;

%% Regularized allocation
H = G.' * G + (rhoT + rhoDelta) * eye(n);
b = G.' * wd + rhoDelta * Tref;
Td = H \ b;

%% Positive tension constraint
for i = 1:n
    if Td(i) < Tmin
        Td(i) = Tmin;
    end
end

end

%% ===== Helpers =====
function q = quat_conj(qin)
q = [qin(1); -qin(2:4)];
end

function q = quat_mult(p,r)
q = [ p(1)*r(1) - p(2:4).'*r(2:4);
      p(1)*r(2:4) + r(1)*p(2:4) + cross(p(2:4),r(2:4)) ];
end
